simulink model "rectificador_pwm"  (R2024a)
settings: Solver=ode23t  StartTime=0.0  StopTime=0.05  FixedStep=sim_sample_time  RelTol=1e-3
values from neighbouring files (symbols this model uses):
  C_filtro_CC = 4 * 470e-6 + 0.47e-6    (= 0.00188047)    [parametros_simulacion.m]
  Ki_Q = 1 / tau_Q    [control_Q.m]
  Kp_Q = Ki_Q * tau_i    [control_Q.m]
  L = 0.5e-3    (= 0.0005)    [parametros_simulacion.m]
  R = 1e-3    (= 0.001)    [parametros_simulacion.m]
  R_load = 30    [parametros_simulacion.m]
  sim_mode = 1    [parametros_simulacion.m]    (also in simulacion.m = 0)
  sim_sample_time = 1e-7    (= 1e-07)    [parametros_simulacion.m]
  Ts = 1 / f_sw    (= 0.0001)    [parametros_simulacion.m]
  Vdc = 300    [parametros_simulacion.m]
  w = 2 * pi * f    (= 314.159265359)    [parametros_simulacion.m]
undefined symbols (not defined in the file or in its folder): ContDC, ContI, Ki, Kp, vgd_step, vgq_step
libraries: spsIGBTDiodeLib x6, slpidlib x5, spsThreePhaseVIMeasurementLib x4, spsSeriesRLCBranchLib x3, spsSVPWMGenerator2LevelLib x2, spsabctoAlphaBetaZeroLib x2, spsdq0toAlphaBetaZeroLib x2, spsDCVoltageSourceLib x1, spsGroundLib x1, spsAlphaBetaZerotoabcLib x1, spsAlphaBetaZerotodq0Lib x1, spsPLL3phLib x1
settings Model: PauseTimes=0.05  Creator=sebar  LastModifiedBy=sebar
settings SolverCC: ZeroCrossAlgorithm=Adaptive  AlgebraicLoopSolver=TrustRegion  DecoupledContinuousIntegration=on
settings DataIOCC: ExternalInput=getinputstruct(op_trim1)  InitialState=steady_state  LimitDataPoints=on  LoadInitialState=on  SaveFinalState=on  SaveFormat=Array  SaveOutput=off  SignalLogging=off  DSMLogging=off  SaveTime=off
settings OptimizationCC: LifeSpan=inf
settings DebuggingCC: ReadBeforeWriteMsg=DisableAll  WriteAfterWriteMsg=DisableAll  WriteAfterReadMsg=DisableAll  IgnoredZcDiagnostic=none  SolverPrmCheckMsg=warning  MultiTaskDSMMsg=none  SFUnexpectedBacktrackingDiag=warning  SFNoUnconditionalDefaultTransitionDiag=warning  SFExecutionAtInitializationDiag=none  ArithmeticOperatorsInVariantConditions=warning
settings HardwareCC: ProdBitPerPointer=32  ProdBitPerSizeT=32  ProdBitPerPtrDiffT=32  ProdLargestAtomicFloat=None  ProdIntDivRoundTo=Undefined  ProdEndianess=Unspecified  ProdWordSize=32  ProdHWDeviceType=32-bit Generic
settings ModelReferenceCC: UpdateModelReferenceTargets=IfOutOfDate  PropagateSignalLabelsOutOfModel=off
settings SFSimCC: SFSimEcho=off  SimUseLocalCustomCode=off  CustomCodeUndefinedFunction=UseInterfaceOnly  SimTargetLang=C++  GPUAcceleration=on  SimDLTargetLibrary=cudnn
settings RTWCC: RTWUseLocalCustomCode=off  GPUComputeCapability=3.5
settings CodeAppCC: StateflowObjectComments=on
settings GRTTargetCC: TargetLangStandard=C89/C90 (ANSI)
settings ConfigComp: CovMetricSettings=dw  CovSaveCumulativeToWorkspaceVar=on  CovSaveSingleToWorkspaceVar=on  CovExternalEMLEnable=off  CovSFcnEnable=off
settings SimscapeCC: SimscapeNormalizeSystem=off

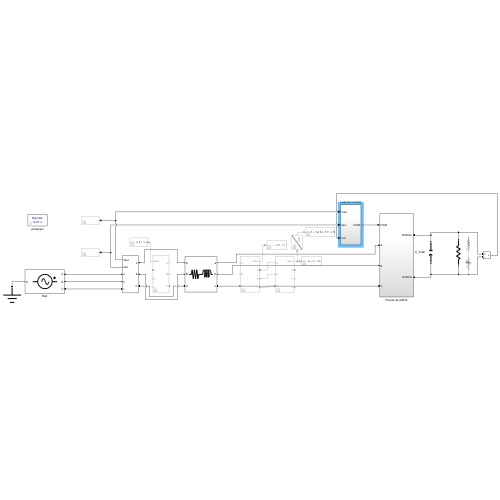
[thumbnail: Simulink's stored preview of the top-level diagram]
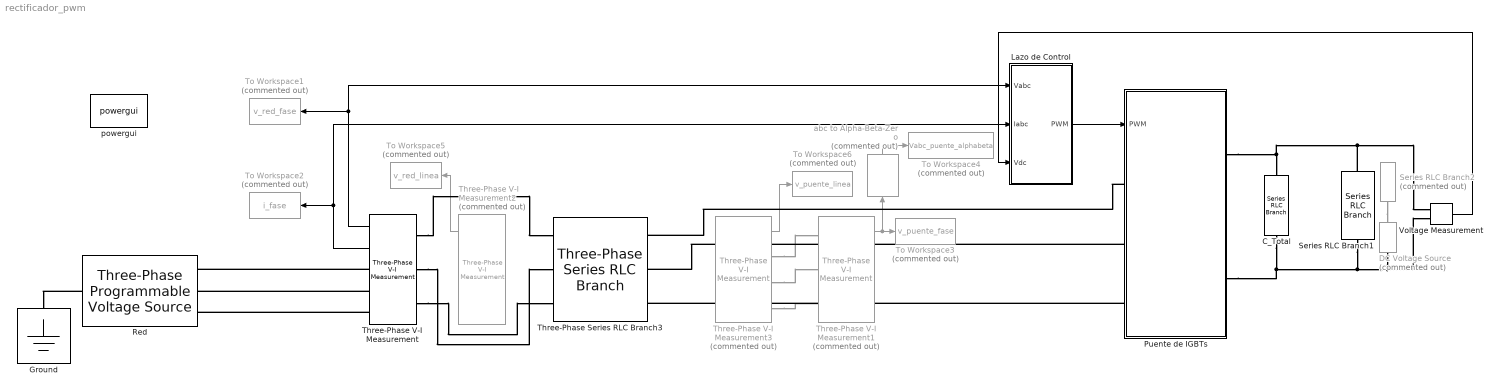
== system rectificador_pwm ==
  C_Total : spsSeriesRLCBranchLib/Series RLC Branch  LConnTagsString=__new0  RConnTagsString=__new0  BranchType=C  Resistance=1  Inductance=1e-3  SetiL0=off  InitialCurrent=0  Capacitance=C_filtro_CC  Setx0=off  InitialVoltage=Vdc*0.75  Measurements=Branch voltage and current
  DC Voltage Source : spsDCVoltageSourceLib/DC Voltage Source  Commented=on  Amplitude=Vdc  Measurements=None
  Ground : spsGroundLib/Ground  LConnTagsString=a
  Lazo de Control : Subsystem
  Puente de IGBTs : Subsystem  VariantControl=Modulacion Senoidal1
  Red : spsThreePhaseProgrammableVoltageSourceLib/Three-Phase Programmable Voltage Source  PositiveSequence="[28*sqrt(3)  0 50]"  VariationEntity=None  VariationType=Table of time-amplitude pairs  VariationTypeAlt=Step  VariationStep=0.5  VariationRate=10  VariationMagnitude=0.3  VariationFrequency=2  VariationTiming=[1 2]  VariationPhaseA=off  Amplitudes=[1 0.8 1.2 1.0]  TimeValues=[0 0.1 0.15 0.2]  HarmonicGeneration=off  HarmonicA=[3 0.2 -25 0]  HarmonicB=[2 0.15 35 2]  Timing="[0.05  3]"  BusType=swing  Pref=0  Qref=0  Qmin=-inf  Qmax=inf
  Series RLC Branch1 : spsSeriesRLCBranchLib/Series RLC Branch  LConnTagsString=__new0  RConnTagsString=__new0  BranchType=R  Resistance=R_load  Inductance=1e-3  SetiL0=off  InitialCurrent=0  Capacitance=1e-6  Setx0=off  InitialVoltage=0  Measurements=None
  Series RLC Branch2 : spsSeriesRLCBranchLib/Series RLC Branch  Commented=on  LConnTagsString=__new0  RConnTagsString=__new0  BranchType=R  Resistance=0.0001  Inductance=1e-3  SetiL0=off  InitialCurrent=0  Capacitance=1e-6  Setx0=off  InitialVoltage=0  Measurements=None
  Three-Phase Series RLC Branch3 : spsThreePhaseSeriesRLCBranchLib/Three-Phase Series RLC Branch  LConnTagsString=A|B|C  RConnTagsString=A|B|C  BranchType=RL  Resistance=R  Inductance=L  Capacitance=1e-6  Measurements=None
  Three-Phase V-I Measurement : spsThreePhaseVIMeasurementLib/Three-Phase V-I Measurement  VoltageMeasurement=phase-to-ground  SetLabelV=off  LabelV=Vabc  Vpu=off  VpuLL=off  CurrentMeasurement=yes  SetLabelI=off  LabelI=Iabc  Ipu=off  Pbase=100e6  Vbase=500e3  OutputType=Complex  PhasorSimulation=off  PSBequivalent=0
  Three-Phase V-I Measurement1 : spsThreePhaseVIMeasurementLib/Three-Phase V-I Measurement  Commented=on  VoltageMeasurement=phase-to-ground  SetLabelV=off  LabelV=Vabc  Vpu=off  VpuLL=off  CurrentMeasurement=no  SetLabelI=off  LabelI=Iabc  Ipu=off  Pbase=100e6  Vbase=500e3  OutputType=Complex  PhasorSimulation=off  PSBequivalent=0
  Three-Phase V-I Measurement2 : spsThreePhaseVIMeasurementLib/Three-Phase V-I Measurement  Commented=on  VoltageMeasurement=phase-to-phase  SetLabelV=off  LabelV=Vabc  Vpu=off  VpuLL=off  CurrentMeasurement=no  SetLabelI=off  LabelI=Iabc  Ipu=off  Pbase=100e6  Vbase=500e3  OutputType=Complex  PhasorSimulation=off  PSBequivalent=0
  Three-Phase V-I Measurement3 : spsThreePhaseVIMeasurementLib/Three-Phase V-I Measurement  Commented=on  VoltageMeasurement=phase-to-phase  SetLabelV=off  LabelV=Vabc  Vpu=off  VpuLL=off  CurrentMeasurement=no  SetLabelI=off  LabelI=Iabc  Ipu=off  Pbase=100e6  Vbase=500e3  OutputType=Complex  PhasorSimulation=off  PSBequivalent=0
  To Workspace1 : ToWorkspace  Commented=on  VariableName=v_red_fase  SaveFormat=Timeseries  SampleTime=-1
  To Workspace2 : ToWorkspace  Commented=on  VariableName=i_fase  SaveFormat=Structure With Time  SampleTime=-1
  To Workspace3 : ToWorkspace  Commented=on  VariableName=v_puente_fase  SaveFormat=Timeseries  SampleTime=-1
  To Workspace4 : ToWorkspace  Commented=on  VariableName=Vabc_puente_alphabeta  SampleTime=-1
  To Workspace5 : ToWorkspace  Commented=on  VariableName=v_red_linea  SaveFormat=Timeseries  SampleTime=-1
  To Workspace6 : ToWorkspace  Commented=on  VariableName=v_puente_linea  SaveFormat=Timeseries  SampleTime=-1
  Voltage Measurement : spsVoltageMeasurementLib/Voltage Measurement  PhasorSimulation=off  OutputType=Complex  PSBequivalent=0
  abc to Alpha-Beta-Zero : spsabctoAlphaBetaZeroLib/abc to Alpha-Beta-Zero  Commented=on
  powergui : sps_lib/powergui  Priority=1  SimulationMode=Discrete  SampleTime=sim_sample_time  frequency=50  Iterations=50  frequencyindice=0  Pbase=100e6  ErrMax=1e-4  UnitsV=kV  UnitsW=MW  buscounter=0  FunctionMessages=off  echomessages=off  EnableUseOfTLC=off  CurrentSourceSwitches=on  DisableSnubberDevices=off  DisableRonSwitches=off  DisableVfSwitches=off  DisplayEquations=off  AutomaticDiscreteSolvers=off  SolverType=Tustin  Interpol=off  ExternalGateDelay=off  methode=on  Ts=100  x0status=blocks  SPID=off  SwTol=0  HookPort=off  NonlinearTolerance=1e-4  nMaxIteration=100  ContinueOnMaxIteration=off  RestoreLinks=warning  ResistiveCurrentMeasurement=off  Frange=[0:2:500]  Ylog=off  Xlog=on  ShowGrid=off  save=off  variable=ZData  structure=0  ZoomFFT=off  StartTime=0.0  cycles=1  DisplayStyle=1  fundamental=60  FreqAxis=off  MaxFrequency=1000  frequencyindicesteady=1  RmsSteady=1  display=off
  wires:
  Voltage Measurement/1 -> Lazo de Control/3(Vdc)
  Three-Phase V-I Measurement/1 -> To Workspace1/1, Lazo de Control/1(Vabc)
  Three-Phase V-I Measurement/2 -> To Workspace2/1, Lazo de Control/2(Iabc)
  Three-Phase V-I Measurement1/1 -> abc to Alpha-Beta-Zero/1, To Workspace3/1
  abc to Alpha-Beta-Zero/1 -> To Workspace4/1
  Three-Phase V-I Measurement2/1 -> To Workspace5/1
  Three-Phase V-I Measurement3/1 -> To Workspace6/1
  Lazo de Control/1(PWM) -> Puente de IGBTs/1(PWM)
  connections:
  Red/LConn1 -- Ground/LConn1
  C_Total/RConn1 -- Series RLC Branch1/RConn1 -- DC Voltage Source/LConn1 -- Voltage Measurement/LConn2 -- Puente de IGBTs/RConn2
  Three-Phase V-I Measurement/RConn1 -- Red/RConn1
  Three-Phase V-I Measurement/RConn2 -- Red/RConn2
  Three-Phase V-I Measurement/RConn3 -- Red/RConn3
  Puente de IGBTs/RConn1 -- Series RLC Branch1/LConn1 -- Voltage Measurement/LConn1 -- C_Total/LConn1
  Series RLC Branch2/RConn1 -- DC Voltage Source/RConn1
  Three-Phase V-I Measurement3/RConn1 -- Three-Phase V-I Measurement1/LConn1
  Three-Phase V-I Measurement3/RConn2 -- Three-Phase V-I Measurement1/LConn2
  Three-Phase V-I Measurement3/RConn3 -- Three-Phase V-I Measurement1/LConn3
  Three-Phase V-I Measurement/LConn1 -- Three-Phase Series RLC Branch3/LConn1
  Three-Phase V-I Measurement/LConn2 -- Three-Phase Series RLC Branch3/LConn2
  Three-Phase V-I Measurement/LConn3 -- Three-Phase Series RLC Branch3/LConn3
  Puente de IGBTs/LConn1 -- Three-Phase Series RLC Branch3/RConn1
  Puente de IGBTs/LConn2 -- Three-Phase Series RLC Branch3/RConn2
  Puente de IGBTs/LConn3 -- Three-Phase Series RLC Branch3/RConn3

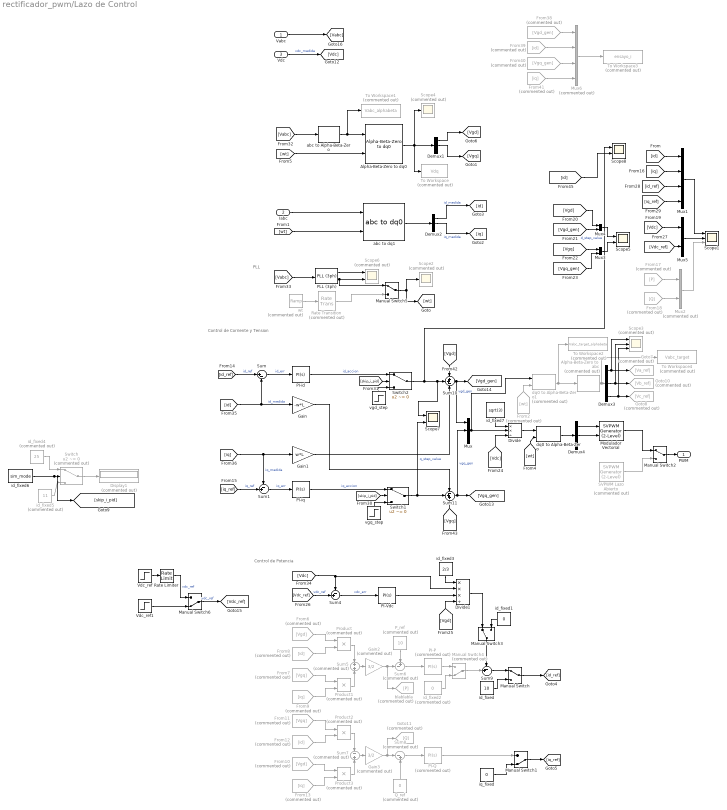
== system rectificador_pwm/Lazo de Control ==
  note: PLL
  note: Control de Potencia
  note: Control de Corriente y Tension
  Vabc : Inport
  Iabc : Inport  Port=2
  Vdc : Inport  Port=3
  Alpha-Beta-Zero to abc : spsAlphaBetaZerotoabcLib/Alpha-Beta-Zero to abc  Commented=on
      settings: LibrarySourceBlock=|
      | sps_lib/Control/Alpha-Beta-Zero
      | to abc
  Alpha-Beta-Zero to dq0 : spsAlphaBetaZerotodq0Lib/Alpha-Beta-Zero to dq0  Alignment=90 degrees behind phase A axis
  Demux{1..4} (4 alike) : Demux  Outputs=3
  Display1 : Display  Commented=on
  Divide : Product  Inputs=**/
  Divide1 : Product  Inputs=***/
  From10 : From  Commented=on  GotoTag=Vgd
  From11 : From  Commented=on  GotoTag=Vgq
  From12 : From  Commented=on  GotoTag=id
  From13 : From  Commented=on  GotoTag=iq
  From17 : From  Commented=on  GotoTag=P
  From18 : From  Commented=on  GotoTag=Q
  From2 : From  Commented=on  GotoTag=wt
  From38 : From  Commented=on  GotoTag=Vgd_gen
  From39 : From  Commented=on  GotoTag=id
  From40 : From  Commented=on  GotoTag=Vgq_gen
  From41 : From  Commented=on  GotoTag=iq
  From6 : From  Commented=on  GotoTag=Vgd
  From7 : From  Commented=on  GotoTag=Vgq
  From8 : From  Commented=on  GotoTag=id
  From9 : From  Commented=on  GotoTag=iq
  Gain : Gain  Gain=-w*L
  Gain1 : Gain  Gain=w*L
  Gain2 : Gain  Commented=on  Gain=3/2
  Gain3 : Gain  Commented=on  Gain=3/2
  Goto10 : Goto  Commented=on  GotoTag=Vb_ref
  Goto11 : Goto  Commented=on  GotoTag=Q
  Goto7 : Goto  Commented=on  GotoTag=Va_ref
  Goto8 : Goto  Commented=on  GotoTag=Vc_ref
  Manual Switch{,2..3,5} (4 alike) : ManualSwitch
  Manual Switch1 : ManualSwitch  CurrentSetting=0
  Manual Switch4 : ManualSwitch  Commented=on  CurrentSetting=0
  Manual Switch6 : ManualSwitch  CurrentSetting=0
  Modulador Vectorial : spsSVPWMGenerator2LevelLib/SVPWM Generator (2-Level)  InputType=alpha-beta components  SwitchingPattern=Pattern #1  Fc=f_sw  ParUref=[0.9144 0 50]  Ts=0
  Mux : Mux  Inputs=3
  Mux1 : Mux
  Mux2 : Mux  Commented=on  Inputs=2
  Mux3 : Mux  Inputs=2
  Mux4 : Mux  Inputs=2
  Mux5 : Mux  Inputs=2
  Mux6 : Mux  Commented=on
  PI-P : slpidlib/PID Controller  Commented=on  Controller=PI  Form=Parallel  TimeDomain=Continuous-time  UseExternalTs=off  SampleTime=1  IntegratorMethod=Forward Euler  FilterMethod=Forward Euler  ControllerParametersSource=internal  P=Kp  I=Ki  UseKiTs=off  D=0  UseExternalDerivativeSource=off  N=100  UseFilter=on  TunerSelectOption=Transfer Function Based (PID Tuner App)  InitialConditionSource=internal  InitialConditionForIntegrator=0  InitialConditionForFilter=0  DifferentiatorICPrevScaledInput=0  ExternalReset=none  TrackingMode=off  Kt=1  LimitOutput=off  SatLimitsSource=internal  UpperSaturationLimit=inf  LowerSaturationLimit=-inf  LinearizeAsGain=on  AntiWindupMode=none  Kb=1  LimitIntegrator=off  UpperIntegratorSaturationLimit=inf  LowerIntegratorSaturationLimit=-inf  POutMin=[]  POutMax=[]  IOutMin=[]  IOutMax=[]  DOutMin=[]  DOutMax=[]  NOutMin=[]  NOutMax=[]  SumOutMin=[]  SumOutMax=[]  SaturationOutMin=[]  SaturationOutMax=[]  PParamMin=[]  PParamMax=[]  IParamMin=[]  IParamMax=[]  DParamMin=[]  DParamMax=[]  NParamMin=[]  NParamMax=[]  KbParamMin=[]  KbParamMax=[]  KtParamMin=[]  KtParamMax=[]  KbOutMin=[]  KbOutMax=[]  KtOutMin=[]  KtOutMax=[]  IntegratorOutMin=[]  IntegratorOutMax=[]  FilterOutMin=[]  FilterOutMax=[]  SumI1OutMin=[]  SumI1OutMax=[]  SumI2OutMin=[]  SumI2OutMax=[]  SumI3OutMin=[]  SumI3OutMax=[]  SumI4OutMin=[]  SumI4OutMax=[]  SumDOutMin=[]  SumDOutMax=[]  DifferentiatorOutMin=[]  DifferentiatorOutMax=[]  FilterDiffOutCoefMin=[]  FilterDiffOutCoefMax=[]  ReciprocalOutMin=[]  ReciprocalOutMax=[]  SumDenOutMin=[]  SumDenOutMax=[]  SumNumOutMin=[]  SumNumOutMax=[]  DivideOutMin=[]  DivideOutMax=[]  UdiffTsProdOutMin=[]  UdiffTsProdOutMax=[]  NTsProdOutMin=[]  NTsProdOutMax=[]  UintegralTsProdOutMin=[]  UintegralTsProdOutMax=[]  UngainTsProdOutMin=[]  UngainTsProdOutMax=[]  ClampingZeroOutDataTypeStr=Inherit: Inherit via back propagation  ClampingZeroOutMin=[]  ClampingZeroOutMax=[]  FilterDenConstantOutDataTypeStr=Inherit: Inherit via back propagation  FilterDenConstantOutMin=[]  FilterDenConstantOutMax=[]  PCopyOutDataTypeStr=Inherit: Inherit via back propagation  PCopyOutMin=[]  PCopyOutMax=[]  NCopyOutDataTypeStr=Inherit: Inherit via back propagation  NCopyOutMin=[]  NCopyOutMax=[]  IntegratorContinuousStateAttributes=''  IntegratorStateMustResolveToSignalObject=off  IntegratorRTWStateStorageClass=Auto  FilterContinuousStateAttributes=''  FilterStateMustResolveToSignalObject=off  FilterRTWStateStorageClass=Auto  ParallelPVariant=InternalParameters  IdealPVariant=Disabled  IVariant=InternalParameters  DVariant=Disabled  IntegratorVariant=Continuous  SatVariant=Disabled  AWVariant=Passthrough  PCopyVariant=Disabled  TRVariant=Disabled  FdbkBlocksVariant=Forward  IdealPFdbkVariant=Disabled  SatFdbkVariant=Disabled  DerivativeFilterVariant=Disabled  NVariant=Disabled  NCopyVariant=Disabled_SignalSpec  FilterICVariant=Disabled  IntegratorICVariant=InternalICs  ExternalResetVariant=Disabled  TRSumVariant=Passthrough  SumFdbkVariant=Disabled  SumVariant=Sum_PI  TsampFilterVariant=InternalTs  TsampNgainVariant=Passthrough  TsampIntegralVariant=Disabled_SignalSpec  ExternalSaturationOutDataTypeStr=Inherit: Same as second input  DerivativeSourceVariant=Disabled
  PI-Q : slpidlib/PID Controller  Commented=on  Controller=PI  Form=Parallel  TimeDomain=Continuous-time  UseExternalTs=off  SampleTime=1  IntegratorMethod=Forward Euler  FilterMethod=Forward Euler  ControllerParametersSource=internal  P=Kp_Q  I=Ki_Q  UseKiTs=off  D=0  UseExternalDerivativeSource=off  N=100  UseFilter=on  TunerSelectOption=Transfer Function Based (PID Tuner App)  InitialConditionSource=internal  InitialConditionForIntegrator=0  InitialConditionForFilter=0  DifferentiatorICPrevScaledInput=0  ExternalReset=none  TrackingMode=off  Kt=1  LimitOutput=off  SatLimitsSource=internal  UpperSaturationLimit=inf  LowerSaturationLimit=-inf  LinearizeAsGain=on  AntiWindupMode=none  Kb=1  LimitIntegrator=off  UpperIntegratorSaturationLimit=inf  LowerIntegratorSaturationLimit=-inf  POutMin=[]  POutMax=[]  IOutMin=[]  IOutMax=[]  DOutMin=[]  DOutMax=[]  NOutMin=[]  NOutMax=[]  SumOutMin=[]  SumOutMax=[]  SaturationOutMin=[]  SaturationOutMax=[]  PParamMin=[]  PParamMax=[]  IParamMin=[]  IParamMax=[]  DParamMin=[]  DParamMax=[]  NParamMin=[]  NParamMax=[]  KbParamMin=[]  KbParamMax=[]  KtParamMin=[]  KtParamMax=[]  KbOutMin=[]  KbOutMax=[]  KtOutMin=[]  KtOutMax=[]  IntegratorOutMin=[]  IntegratorOutMax=[]  FilterOutMin=[]  FilterOutMax=[]  SumI1OutMin=[]  SumI1OutMax=[]  SumI2OutMin=[]  SumI2OutMax=[]  SumI3OutMin=[]  SumI3OutMax=[]  SumI4OutMin=[]  SumI4OutMax=[]  SumDOutMin=[]  SumDOutMax=[]  DifferentiatorOutMin=[]  DifferentiatorOutMax=[]  FilterDiffOutCoefMin=[]  FilterDiffOutCoefMax=[]  ReciprocalOutMin=[]  ReciprocalOutMax=[]  SumDenOutMin=[]  SumDenOutMax=[]  SumNumOutMin=[]  SumNumOutMax=[]  DivideOutMin=[]  DivideOutMax=[]  UdiffTsProdOutMin=[]  UdiffTsProdOutMax=[]  NTsProdOutMin=[]  NTsProdOutMax=[]  UintegralTsProdOutMin=[]  UintegralTsProdOutMax=[]  UngainTsProdOutMin=[]  UngainTsProdOutMax=[]  ClampingZeroOutDataTypeStr=Inherit: Inherit via back propagation  ClampingZeroOutMin=[]  ClampingZeroOutMax=[]  FilterDenConstantOutDataTypeStr=Inherit: Inherit via back propagation  FilterDenConstantOutMin=[]  FilterDenConstantOutMax=[]  PCopyOutDataTypeStr=Inherit: Inherit via back propagation  PCopyOutMin=[]  PCopyOutMax=[]  NCopyOutDataTypeStr=Inherit: Inherit via back propagation  NCopyOutMin=[]  NCopyOutMax=[]  IntegratorContinuousStateAttributes=''  IntegratorStateMustResolveToSignalObject=off  IntegratorRTWStateStorageClass=Auto  FilterContinuousStateAttributes=''  FilterStateMustResolveToSignalObject=off  FilterRTWStateStorageClass=Auto  ParallelPVariant=InternalParameters  IdealPVariant=Disabled  IVariant=InternalParameters  DVariant=Disabled  IntegratorVariant=Continuous  SatVariant=Disabled  AWVariant=Passthrough  PCopyVariant=Disabled  TRVariant=Disabled  FdbkBlocksVariant=Forward  IdealPFdbkVariant=Disabled  SatFdbkVariant=Disabled  DerivativeFilterVariant=Disabled  NVariant=Disabled  NCopyVariant=Disabled_SignalSpec  FilterICVariant=Disabled  IntegratorICVariant=InternalICs  ExternalResetVariant=Disabled  TRSumVariant=Passthrough  SumFdbkVariant=Disabled  SumVariant=Sum_PI  TsampFilterVariant=InternalTs  TsampNgainVariant=Passthrough  TsampIntegralVariant=Disabled_SignalSpec  ExternalSaturationOutDataTypeStr=Inherit: Same as second input  DerivativeSourceVariant=Disabled
  PI-Vdc : slpidlib/PID Controller  Controller=PI  Form=Parallel  TimeDomain=Continuous-time  UseExternalTs=off  SampleTime=1  IntegratorMethod=Forward Euler  FilterMethod=Forward Euler  ControllerParametersSource=internal  P=ContDC.Kp  I=ContDC.Ki  UseKiTs=off  D=0  UseExternalDerivativeSource=off  N=100  UseFilter=on  TunerSelectOption=Transfer Function Based (PID Tuner App)  InitialConditionSource=internal  InitialConditionForIntegrator=0  InitialConditionForFilter=0  DifferentiatorICPrevScaledInput=0  ExternalReset=none  TrackingMode=off  Kt=1  LimitOutput=off  SatLimitsSource=internal  UpperSaturationLimit=inf  LowerSaturationLimit=-inf  LinearizeAsGain=on  AntiWindupMode=none  Kb=1  LimitIntegrator=off  UpperIntegratorSaturationLimit=inf  LowerIntegratorSaturationLimit=-inf  POutMin=[]  POutMax=[]  IOutMin=[]  IOutMax=[]  DOutMin=[]  DOutMax=[]  NOutMin=[]  NOutMax=[]  SumOutMin=[]  SumOutMax=[]  SaturationOutMin=[]  SaturationOutMax=[]  PParamMin=[]  PParamMax=[]  IParamMin=[]  IParamMax=[]  DParamMin=[]  DParamMax=[]  NParamMin=[]  NParamMax=[]  KbParamMin=[]  KbParamMax=[]  KtParamMin=[]  KtParamMax=[]  KbOutMin=[]  KbOutMax=[]  KtOutMin=[]  KtOutMax=[]  IntegratorOutMin=[]  IntegratorOutMax=[]  FilterOutMin=[]  FilterOutMax=[]  SumI1OutMin=[]  SumI1OutMax=[]  SumI2OutMin=[]  SumI2OutMax=[]  SumI3OutMin=[]  SumI3OutMax=[]  SumI4OutMin=[]  SumI4OutMax=[]  SumDOutMin=[]  SumDOutMax=[]  DifferentiatorOutMin=[]  DifferentiatorOutMax=[]  FilterDiffOutCoefMin=[]  FilterDiffOutCoefMax=[]  ReciprocalOutMin=[]  ReciprocalOutMax=[]  SumDenOutMin=[]  SumDenOutMax=[]  SumNumOutMin=[]  SumNumOutMax=[]  DivideOutMin=[]  DivideOutMax=[]  UdiffTsProdOutMin=[]  UdiffTsProdOutMax=[]  NTsProdOutMin=[]  NTsProdOutMax=[]  UintegralTsProdOutMin=[]  UintegralTsProdOutMax=[]  UngainTsProdOutMin=[]  UngainTsProdOutMax=[]  ClampingZeroOutDataTypeStr=Inherit: Inherit via back propagation  ClampingZeroOutMin=[]  ClampingZeroOutMax=[]  FilterDenConstantOutDataTypeStr=Inherit: Inherit via back propagation  FilterDenConstantOutMin=[]  FilterDenConstantOutMax=[]  PCopyOutDataTypeStr=Inherit: Inherit via back propagation  PCopyOutMin=[]  PCopyOutMax=[]  NCopyOutDataTypeStr=Inherit: Inherit via back propagation  NCopyOutMin=[]  NCopyOutMax=[]  IntegratorContinuousStateAttributes=''  IntegratorStateMustResolveToSignalObject=off  IntegratorRTWStateStorageClass=Auto  FilterContinuousStateAttributes=''  FilterStateMustResolveToSignalObject=off  FilterRTWStateStorageClass=Auto  ParallelPVariant=InternalParameters  IdealPVariant=Disabled  IVariant=InternalParameters  DVariant=Disabled  IntegratorVariant=Continuous  SatVariant=Disabled  AWVariant=Passthrough  PCopyVariant=Disabled  TRVariant=Disabled  FdbkBlocksVariant=Forward  IdealPFdbkVariant=Disabled  SatFdbkVariant=Disabled  DerivativeFilterVariant=Disabled  NVariant=Disabled  NCopyVariant=Disabled_SignalSpec  FilterICVariant=Disabled  IntegratorICVariant=InternalICs  ExternalResetVariant=Disabled  TRSumVariant=Passthrough  SumFdbkVariant=Disabled  SumVariant=Sum_PI  TsampFilterVariant=InternalTs  TsampNgainVariant=Passthrough  TsampIntegralVariant=Disabled_SignalSpec  ExternalSaturationOutDataTypeStr=Inherit: Same as second input  DerivativeSourceVariant=Disabled
  PI-id : slpidlib/PID Controller  Controller=PI  Form=Parallel  TimeDomain=Continuous-time  UseExternalTs=off  SampleTime=1  IntegratorMethod=Forward Euler  FilterMethod=Forward Euler  ControllerParametersSource=internal  P=ContI.Kp  I=ContI.Ki  UseKiTs=off  D=0  UseExternalDerivativeSource=off  N=100  UseFilter=on  TunerSelectOption=Transfer Function Based (PID Tuner App)  InitialConditionSource=internal  InitialConditionForIntegrator=0  InitialConditionForFilter=0  DifferentiatorICPrevScaledInput=0  ExternalReset=none  TrackingMode=off  Kt=1  LimitOutput=off  SatLimitsSource=internal  UpperSaturationLimit=20  LowerSaturationLimit=-20  LinearizeAsGain=on  AntiWindupMode=none  Kb=1  LimitIntegrator=off  UpperIntegratorSaturationLimit=inf  LowerIntegratorSaturationLimit=-inf  POutMin=[]  POutMax=[]  IOutMin=[]  IOutMax=[]  DOutMin=[]  DOutMax=[]  NOutMin=[]  NOutMax=[]  SumOutMin=[]  SumOutMax=[]  SaturationOutMin=[]  SaturationOutMax=[]  PParamMin=[]  PParamMax=[]  IParamMin=[]  IParamMax=[]  DParamMin=[]  DParamMax=[]  NParamMin=[]  NParamMax=[]  KbParamMin=[]  KbParamMax=[]  KtParamMin=[]  KtParamMax=[]  KbOutMin=[]  KbOutMax=[]  KtOutMin=[]  KtOutMax=[]  IntegratorOutMin=[]  IntegratorOutMax=[]  FilterOutMin=[]  FilterOutMax=[]  SumI1OutMin=[]  SumI1OutMax=[]  SumI2OutMin=[]  SumI2OutMax=[]  SumI3OutMin=[]  SumI3OutMax=[]  SumI4OutMin=[]  SumI4OutMax=[]  SumDOutMin=[]  SumDOutMax=[]  DifferentiatorOutMin=[]  DifferentiatorOutMax=[]  FilterDiffOutCoefMin=[]  FilterDiffOutCoefMax=[]  ReciprocalOutMin=[]  ReciprocalOutMax=[]  SumDenOutMin=[]  SumDenOutMax=[]  SumNumOutMin=[]  SumNumOutMax=[]  DivideOutMin=[]  DivideOutMax=[]  UdiffTsProdOutMin=[]  UdiffTsProdOutMax=[]  NTsProdOutMin=[]  NTsProdOutMax=[]  UintegralTsProdOutMin=[]  UintegralTsProdOutMax=[]  UngainTsProdOutMin=[]  UngainTsProdOutMax=[]  ClampingZeroOutDataTypeStr=Inherit: Inherit via back propagation  ClampingZeroOutMin=[]  ClampingZeroOutMax=[]  FilterDenConstantOutDataTypeStr=Inherit: Inherit via back propagation  FilterDenConstantOutMin=[]  FilterDenConstantOutMax=[]  PCopyOutDataTypeStr=Inherit: Inherit via back propagation  PCopyOutMin=[]  PCopyOutMax=[]  NCopyOutDataTypeStr=Inherit: Inherit via back propagation  NCopyOutMin=[]  NCopyOutMax=[]  IntegratorContinuousStateAttributes=''  IntegratorStateMustResolveToSignalObject=off  IntegratorRTWStateStorageClass=Auto  FilterContinuousStateAttributes=''  FilterStateMustResolveToSignalObject=off  FilterRTWStateStorageClass=Auto  ParallelPVariant=InternalParameters  IdealPVariant=Disabled  IVariant=InternalParameters  DVariant=Disabled  IntegratorVariant=Continuous  SatVariant=Disabled  AWVariant=Passthrough  PCopyVariant=Disabled  TRVariant=Disabled  FdbkBlocksVariant=Forward  IdealPFdbkVariant=Disabled  SatFdbkVariant=Disabled  DerivativeFilterVariant=Disabled  NVariant=Disabled  NCopyVariant=Disabled_SignalSpec  FilterICVariant=Disabled  IntegratorICVariant=InternalICs  ExternalResetVariant=Disabled  TRSumVariant=Passthrough  SumFdbkVariant=Disabled  SumVariant=Sum_PI  TsampFilterVariant=InternalTs  TsampNgainVariant=Passthrough  TsampIntegralVariant=Disabled_SignalSpec  ExternalSaturationOutDataTypeStr=Inherit: Same as second input  DerivativeSourceVariant=Disabled
  PI-iq : slpidlib/PID Controller  Controller=PI  Form=Parallel  TimeDomain=Continuous-time  UseExternalTs=off  SampleTime=1  IntegratorMethod=Forward Euler  FilterMethod=Forward Euler  ControllerParametersSource=internal  P=ContI.Kp  I=ContI.Ki  UseKiTs=off  D=0  UseExternalDerivativeSource=off  N=100  UseFilter=on  TunerSelectOption=Transfer Function Based (PID Tuner App)  InitialConditionSource=internal  InitialConditionForIntegrator=0  InitialConditionForFilter=0  DifferentiatorICPrevScaledInput=0  ExternalReset=none  TrackingMode=off  Kt=1  LimitOutput=off  SatLimitsSource=internal  UpperSaturationLimit=20  LowerSaturationLimit=-20  LinearizeAsGain=on  AntiWindupMode=none  Kb=1  LimitIntegrator=off  UpperIntegratorSaturationLimit=inf  LowerIntegratorSaturationLimit=-inf  POutMin=[]  POutMax=[]  IOutMin=[]  IOutMax=[]  DOutMin=[]  DOutMax=[]  NOutMin=[]  NOutMax=[]  SumOutMin=[]  SumOutMax=[]  SaturationOutMin=[]  SaturationOutMax=[]  PParamMin=[]  PParamMax=[]  IParamMin=[]  IParamMax=[]  DParamMin=[]  DParamMax=[]  NParamMin=[]  NParamMax=[]  KbParamMin=[]  KbParamMax=[]  KtParamMin=[]  KtParamMax=[]  KbOutMin=[]  KbOutMax=[]  KtOutMin=[]  KtOutMax=[]  IntegratorOutMin=[]  IntegratorOutMax=[]  FilterOutMin=[]  FilterOutMax=[]  SumI1OutMin=[]  SumI1OutMax=[]  SumI2OutMin=[]  SumI2OutMax=[]  SumI3OutMin=[]  SumI3OutMax=[]  SumI4OutMin=[]  SumI4OutMax=[]  SumDOutMin=[]  SumDOutMax=[]  DifferentiatorOutMin=[]  DifferentiatorOutMax=[]  FilterDiffOutCoefMin=[]  FilterDiffOutCoefMax=[]  ReciprocalOutMin=[]  ReciprocalOutMax=[]  SumDenOutMin=[]  SumDenOutMax=[]  SumNumOutMin=[]  SumNumOutMax=[]  DivideOutMin=[]  DivideOutMax=[]  UdiffTsProdOutMin=[]  UdiffTsProdOutMax=[]  NTsProdOutMin=[]  NTsProdOutMax=[]  UintegralTsProdOutMin=[]  UintegralTsProdOutMax=[]  UngainTsProdOutMin=[]  UngainTsProdOutMax=[]  ClampingZeroOutDataTypeStr=Inherit: Inherit via back propagation  ClampingZeroOutMin=[]  ClampingZeroOutMax=[]  FilterDenConstantOutDataTypeStr=Inherit: Inherit via back propagation  FilterDenConstantOutMin=[]  FilterDenConstantOutMax=[]  PCopyOutDataTypeStr=Inherit: Inherit via back propagation  PCopyOutMin=[]  PCopyOutMax=[]  NCopyOutDataTypeStr=Inherit: Inherit via back propagation  NCopyOutMin=[]  NCopyOutMax=[]  IntegratorContinuousStateAttributes=''  IntegratorStateMustResolveToSignalObject=off  IntegratorRTWStateStorageClass=Auto  FilterContinuousStateAttributes=''  FilterStateMustResolveToSignalObject=off  FilterRTWStateStorageClass=Auto  ParallelPVariant=InternalParameters  IdealPVariant=Disabled  IVariant=InternalParameters  DVariant=Disabled  IntegratorVariant=Continuous  SatVariant=Disabled  AWVariant=Passthrough  PCopyVariant=Disabled  TRVariant=Disabled  FdbkBlocksVariant=Forward  IdealPFdbkVariant=Disabled  SatFdbkVariant=Disabled  DerivativeFilterVariant=Disabled  NVariant=Disabled  NCopyVariant=Disabled_SignalSpec  FilterICVariant=Disabled  IntegratorICVariant=InternalICs  ExternalResetVariant=Disabled  TRSumVariant=Passthrough  SumFdbkVariant=Disabled  SumVariant=Sum_PI  TsampFilterVariant=InternalTs  TsampNgainVariant=Passthrough  TsampIntegralVariant=Disabled_SignalSpec  ExternalSaturationOutDataTypeStr=Inherit: Same as second input  DerivativeSourceVariant=Disabled
  PLL (3ph) : spsPLL3phLib/PLL (3ph)  Fmin=45  Par_Init=[0, 50]  ParK=[180, 3200, 1]  TcD=1e-4  MaxRateChangeFreq=12  FilterCutOffFreq=25  Ts=Ts  AGC=on
  P_ref : Constant  Commented=on  Value=10
  Product{,1..3} (4 alike) : Product  Commented=on
  Q_ref : Constant  Commented=on  Value=0
  Rate Limiter : RateLimiter  RisingSlewLimit=1000  FallingSlewLimit=-1000
  Rate Transition : RateTransition  Commented=on
  SVPWM Lazo Abierto : spsSVPWMGenerator2LevelLib/SVPWM Generator (2-Level)  Commented=on  InputType=Internally generated  SwitchingPattern=Pattern #1  Fc=2000  ParUref=[0.9144 0 50]  Ts=0
  Scope1 : Scope  NumInputPorts=3
  Scope2 : Scope  Commented=on
  Scope3 : Scope  Commented=on  NumInputPorts=3
  Scope4 : Scope  Commented=on
  Scope5 : Scope  NumInputPorts=2
  Scope6 : Scope  Commented=on  NumInputPorts=2
  Scope7 : Scope  NumInputPorts=2
  Scope8 : Scope  NumInputPorts=2
  Sum : Sum  Inputs=|+-
  Sum1 : Sum  Inputs=-+|
  Sum10 : Sum  Inputs=++-
  Sum11 : Sum  Inputs=-++
  Sum4 : Sum  Inputs=-+|
  Sum5 : Sum  Commented=on  Inputs=+|+
  Sum6 : Sum  Commented=on  Inputs=+-|
  Sum7 : Sum  Commented=on  Inputs=-|+
  Sum8 : Sum  Commented=on  Inputs=|-+
  Sum9 : Sum  Inputs=-+|
  Switch : Switch  Commented=on  Criteria=u2 ~= 0  SaturateOnIntegerOverflow=off  InputSameDT=off
  Switch1 : Switch  Criteria=u2 ~= 0  SaturateOnIntegerOverflow=off  InputSameDT=off
  Switch2 : Switch  Criteria=u2 ~= 0  SaturateOnIntegerOverflow=off  InputSameDT=off
  To Workspace : ToWorkspace  Commented=on  VariableName=Vdq  SaveFormat=Timeseries  SampleTime=-1
  To Workspace1 : ToWorkspace  Commented=on  VariableName=Vabc_alphabeta  SampleTime=-1
      settings: Save2DSignal=2-D array (concatenate along first dimension)
  To Workspace2 : ToWorkspace  Commented=on  VariableName=Vabc_target_alphabeta  SaveFormat=Structure With Time  SampleTime=-1
      settings: Save2DSignal=2-D array (concatenate along first dimension)
  To Workspace3 : ToWorkspace  Commented=on  VariableName=ensayo_i  SaveFormat=Timeseries  SampleTime=-1
  To Workspace4 : ToWorkspace  Commented=on  VariableName=Vabc_target  SaveFormat=Structure With Time  SampleTime=-1
      settings: Save2DSignal=2-D array (concatenate along first dimension)
  Vdc_ref : Step  Time=0.05  After=Vdc  SampleTime=0
  Vdc_ref1 : Step  Time=0.05  Before=Vdc  After=Vdc  SampleTime=0
  abc to Alpha-Beta-Zero : spsabctoAlphaBetaZeroLib/abc to Alpha-Beta-Zero
  abc to dq1 : spsabctodq0Lib/abc to dq0  Alignment=90 degrees behind phase A axis
  blablabla : Goto  Commented=on  GotoTag=P
  dq0 to Alpha-Beta-Zero : spsdq0toAlphaBetaZeroLib/dq0 to Alpha-Beta-Zero  Alignment=90 degrees behind phase A axis
  dq0 to Alpha-Beta-Zero1 : spsdq0toAlphaBetaZeroLib/dq0 to Alpha-Beta-Zero  Commented=on  Alignment=90 degrees behind phase A axis
  id_fixed : Constant  Value=10
  id_fixed1 : Constant  Value=0
  id_fixed2 : Constant  Commented=on  Value=0
  id_fixed3 : Constant  Value=2/3
  id_fixed4 : Constant  Commented=on  Value=25
  id_fixed5 : Constant  Commented=on  Value=11
  id_fixed6 : Constant  Value=sim_mode
  id_fixed7 : Constant  Value=sqrt(3)
  iq_fixed : Constant  Value=0
  vgd_step : Step  Time=vgd_step.time  Before=vgd_step.start_value  After=vgd_step.end_value  SampleTime=1e-5
  vgq_step : Step  Time=vgq_step.time  Before=vgq_step.start_value  After=vgq_step.start_value*(1+vgq_step.percentage/100)  SampleTime=1e-5
  wt : simulink/Sources/Ramp  Commented=on  slope=2*pi*50  start=0  InitialOutput=0
  PWM : Outport
  wires:
  Manual Switch2/1 -> PWM/1
  [wt] -> Alpha-Beta-Zero to dq0/2
  Vabc/1 -> [Vabc]
  [wt] -> abc to dq1/2
  Iabc/1 -> abc to dq1/1
  Alpha-Beta-Zero to dq0/1 -> Scope4/1, To Workspace/1, Demux1/1
  Demux1/1 -> [Vgd]
  Demux1/2 -> [Vgq]
  abc to dq1/1 -> Demux2/1
  [id] -> Gain/1, Sum/2  "id_medida"
  [iq] -> Gain1/1, Sum1/1  "iq_medida"
  [id_ref] -> Sum/1  "id_ref"
  [iq_ref] -> Sum1/2  "iq_ref"
  Sum/1 -> PI-id/1  "id_err"
  Sum1/1 -> PI-iq/1  "iq_err"
  Gain1/1 -> Sum10/3
  PI-iq/1 -> Switch1/1  "iq_accion"
  Gain/1 -> Sum11/1
  Sum11/1 -> [Vgq_gen], Mux/2  "vgq_gen"
  [wt] -> dq0 to Alpha-Beta-Zero/2
  Alpha-Beta-Zero to abc/1 -> To Workspace4/1, Demux3/1
  Demux3/1 -> Goto7/1, Scope3/1
  Demux3/2 -> Goto10/1, Scope3/2
  Demux3/3 -> Goto8/1, Scope3/3
  Vdc/1 -> [Vdc]  "vdc_medida"
  [Vdc_ref] -> Sum4/2  "vdc_ref"
  Sum4/1 -> PI-Vdc/1  "vdc_err"
  From8/1 -> Product/2
  From6/1 -> Product/1
  From7/1 -> Product1/1
  From9/1 -> Product1/2
  Product/1 -> Sum5/1
  Product1/1 -> Sum5/2
  Gain2/1 -> Sum6/2, blablabla/1
  P_ref/1 -> Sum6/1
  From12/1 -> Product2/2
  From13/1 -> Product3/2
  Product2/1 -> Sum7/1
  Product3/1 -> Sum7/2
  Gain3/1 -> Sum8/1, Goto11/1
  Q_ref/1 -> Sum8/2
  From10/1 -> Product3/1
  From11/1 -> Product2/1
  Sum6/1 -> PI-P/1
  Sum8/1 -> PI-Q/1
  PI-P/1 -> Manual Switch4/1
  abc to Alpha-Beta-Zero/1 -> To Workspace1/1, Alpha-Beta-Zero to dq0/1
  dq0 to Alpha-Beta-Zero/1 -> Demux4/1
  Demux4/1 -> Modulador Vectorial/1
  Demux4/2 -> Modulador Vectorial/2
  Sum9/1 -> Manual Switch/1
  id_fixed/1 -> Manual Switch/2
  PI-Q/1 -> Manual Switch1/1
  iq_fixed/1 -> Manual Switch1/2
  Manual Switch1/1 -> [iq_ref]
  Modulador Vectorial/1 -> Manual Switch2/1
  SVPWM Lazo Abierto/1 -> Manual Switch2/2
  Manual Switch3/1 -> Sum9/1
  id_fixed1/1 -> Manual Switch3/2
  From17/1 -> Mux2/1
  From18/1 -> Mux2/2
  [iq] -> Mux1/2
  [id] -> Mux1/1
  [Vdc] -> Mux5/1
  Mux1/1 -> Scope1/1
  Mux2/1 -> Scope1/3
  Mux3/1 -> Scope5/2
  Mux4/1 -> Scope5/1
  id_fixed2/1 -> Manual Switch4/2
  Manual Switch4/1 -> Sum9/2
  [Vgd_gen] -> Mux4/2
  [Vgd] -> Mux4/1
  [Vgq] -> Mux3/1
  [Vgq_gen] -> Mux3/2
  wt/1 -> Rate Transition/1
  Manual Switch5/1 -> [wt], Scope2/1
  PLL (3ph)/2 -> Scope6/2, Manual Switch5/1
  Rate Transition/1 -> Manual Switch5/2
  PLL (3ph)/1 -> Scope6/1
  [Vdc] -> Divide/3
  Sum5/1 -> Gain2/1
  Sum7/1 -> Gain3/1
  PI-Vdc/1 -> Divide1/3
  [Vgd] -> Divide1/4
  Divide1/1 -> Manual Switch3/1
  Divide/1 -> dq0 to Alpha-Beta-Zero/1
  Mux/1 -> dq0 to Alpha-Beta-Zero1/1, Divide/2
  Vdc_ref/1 -> Rate Limiter/1
  Manual Switch6/1 -> [Vdc_ref]  "vdc_ref"
  Mux5/1 -> Scope1/2
  [Vdc_ref] -> Mux5/2
  [id_ref] -> Mux1/3
  [iq_ref] -> Mux1/4
  Manual Switch/1 -> [id_ref]
  id_fixed4/1 -> Switch/1
  id_fixed5/1 -> Switch/3
  Switch/1 -> Display1/1
  [skip_i_pid] -> Switch1/2
  [skip_i_pid] -> Switch2/2
  PI-id/1 -> Switch2/1  "id_accion"
  [Vabc] -> abc to Alpha-Beta-Zero/1
  [Vabc] -> PLL (3ph)/1
  [Vdc] -> Divide1/2, Sum4/1
  Demux2/1 -> [id]  "id_medida"
  Demux2/2 -> [iq]  "iq_medida"
  id_fixed6/1 -> [skip_i_pid], Switch/2
  Sum10/1 -> [Vgd_gen], Mux/1  "vgd_gen"
  vgd_step/1 -> Switch2/3
  vgq_step/1 -> Switch1/3
  Mux6/1 -> To Workspace3/1
  From38/1 -> Mux6/1
  From39/1 -> Mux6/2
  From40/1 -> Mux6/3
  From41/1 -> Mux6/4
  Rate Limiter/1 -> Manual Switch6/1  "vdc_ref"
  Vdc_ref1/1 -> Manual Switch6/2
  Switch2/1 -> Scope8/1, Scope7/1, Sum10/2  "d_step_value"
  [Vgd] -> Sum10/1
  Switch1/1 -> Scope7/2, Sum11/2  "q_step_value"
  [Vgq] -> Sum11/3
  From2/1 -> dq0 to Alpha-Beta-Zero1/2
  dq0 to Alpha-Beta-Zero1/1 -> Alpha-Beta-Zero to abc/1, To Workspace2/1
  id_fixed3/1 -> Divide1/1
  id_fixed7/1 -> Divide/1
  [id] -> Scope8/2

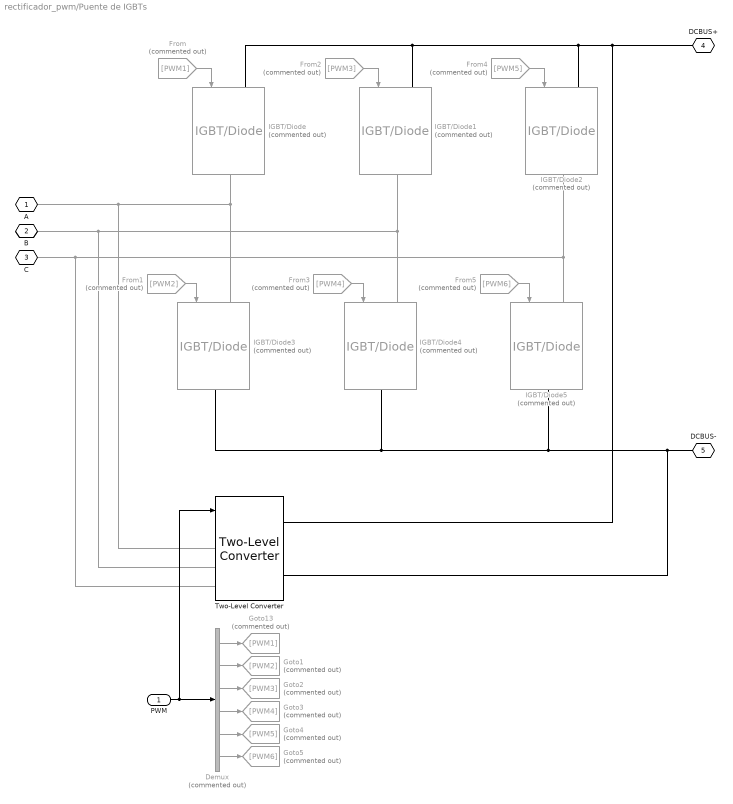
== system rectificador_pwm/Puente de IGBTs ==
  PWM : Inport
  Demux : Demux  Commented=on  Outputs=6
  From : From  Commented=on  GotoTag=PWM1
  From1 : From  Commented=on  GotoTag=PWM2
  From2 : From  Commented=on  GotoTag=PWM3
  From3 : From  Commented=on  GotoTag=PWM4
  From4 : From  Commented=on  GotoTag=PWM5
  From5 : From  Commented=on  GotoTag=PWM6
  Goto1 : Goto  Commented=on  GotoTag=PWM2
  Goto13 : Goto  Commented=on  GotoTag=PWM1
  Goto2 : Goto  Commented=on  GotoTag=PWM3
  Goto3 : Goto  Commented=on  GotoTag=PWM4
  Goto4 : Goto  Commented=on  GotoTag=PWM5
  Goto5 : Goto  Commented=on  GotoTag=PWM6
  IGBT/Diode{,1..5} (6 alike) : spsIGBTDiodeLib/IGBT//Diode  Commented=on  Ron=ron  Rs=Rs  Cs=Cs  Measurements=off
  Two-Level Converter : spsTwoLevelConverterLib/Two-Level Converter  ModelType=Switching devices  Ron=ron  Rs=Rs  Cs=Cs  Vforward=[0,0]  Ron_Diode=1e-3  Rs_Diode=1e6  Cs_Diode=inf  Vf_Diode=1e-3  Rs_CurrentSource=inf  Ron_ACsource=1e-3
      settings: LibrarySourceBlock=sps_lib/Power Electronics/Two-Level Converter
  A : PMIOPort  Tag=PMCPort  Side=Left
  B : PMIOPort  Tag=PMCPort  Port=2  Side=Left
  C : PMIOPort  Tag=PMCPort  Port=3  Side=Left
  DCBUS+ : PMIOPort  Tag=PMCPort  Port=4  Side=Right
  DCBUS- : PMIOPort  Tag=PMCPort  Port=5  Side=Right
  wires:
  PWM/1 -> Two-Level Converter/1, Demux/1
  Demux/1 -> Goto13/1
  Demux/2 -> Goto1/1
  Demux/3 -> Goto2/1
  Demux/4 -> Goto3/1
  Demux/5 -> Goto4/1
  Demux/6 -> Goto5/1
  From1/1 -> IGBT/Diode3/1
  From3/1 -> IGBT/Diode4/1
  From5/1 -> IGBT/Diode5/1
  From/1 -> IGBT/Diode/1
  From2/1 -> IGBT/Diode1/1
  From4/1 -> IGBT/Diode2/1
  connections:
  IGBT/Diode/RConn1 -- A/RConn1 -- Two-Level Converter/LConn1 -- IGBT/Diode3/LConn1
  IGBT/Diode1/RConn1 -- B/RConn1 -- Two-Level Converter/LConn2 -- IGBT/Diode4/LConn1
  IGBT/Diode2/RConn1 -- C/RConn1 -- Two-Level Converter/LConn3 -- IGBT/Diode5/LConn1
  DCBUS+/RConn1 -- Two-Level Converter/RConn1 -- IGBT/Diode2/LConn1 -- IGBT/Diode1/LConn1 -- IGBT/Diode/LConn1
  IGBT/Diode4/RConn1 -- IGBT/Diode3/RConn1 -- Two-Level Converter/RConn2 -- DCBUS-/RConn1 -- IGBT/Diode5/RConn1
